simulink model "Simulation_DC_Motor"  (R2024b)
settings: Solver=VariableStepAuto  StartTime=0.0  StopTime=10.0  RelTol=1e-3
model workspace (MAT data in the model file):
  Cm = 38.2
  J = 0.012
  La = 0.004
  Ra = 0.25
  phi = 0.04
settings Model: Creator=arthu  LastModifiedBy=arthu

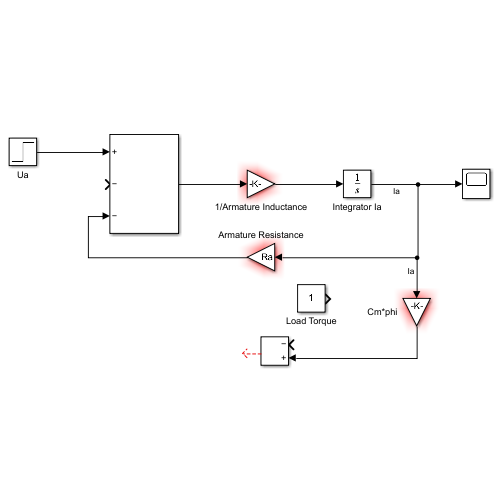
[thumbnail: Simulink's stored preview of the top-level diagram]
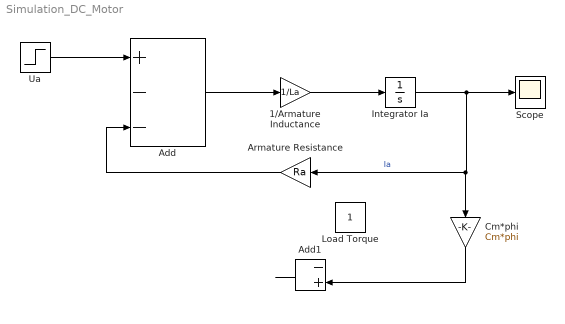
== system Simulation_DC_Motor ==
  1/Armature Inductance : Gain  Gain=1/La
  Add : Sum  Inputs=+--
  Add1 : Sum  Inputs=-+
  Armature Resistance : Gain  Gain=Ra
  Cm*phi : Gain  Gain=Cm*phi
  Integrator Ia : Integrator
  Load Torque : Constant
  Scope : Scope
  Ua : Step  Time=0.02  After=20  SampleTime=0
  wires:
  Ua/1 -> Add/1
  Add/1 -> 1/Armature Inductance/1
  1/Armature Inductance/1 -> Integrator Ia/1
  Integrator Ia/1 -> Cm*phi/1, Armature Resistance/1, Scope/1  "Ia"
  Armature Resistance/1 -> Add/3
  Cm*phi/1 -> Add1/2
  Add1/1 -> ?
